simulink model "engine_approxdyn"  (Simulink 7.2)
settings: Solver=ode3  StartTime=0.0  StopTime=10.0  FixedStep=0.02  RelTol=1e-3
settings Model: Creator=E183308  LastModifiedBy=E183308

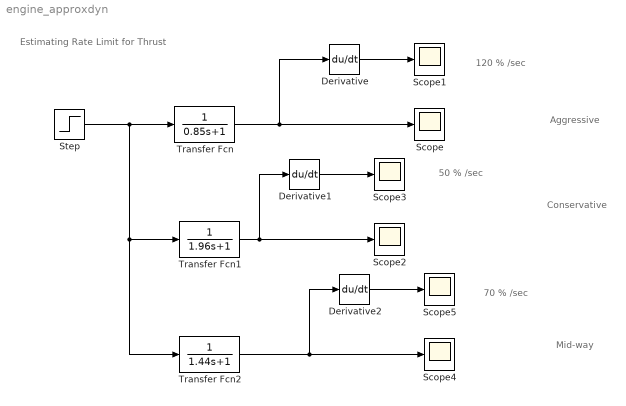
== system engine_approxdyn ==
  note: Conservative
  note: Estimating Rate Limit
      | for Thrust
  note: Aggressive
  note: Mid-way
  note: 120 % /sec
  note: 50 % /sec
  note: 70 % /sec
  Derivative : Derivative
  Derivative1 : Derivative
  Derivative2 : Derivative
  Scope{,1..5} (6 alike) : Scope
      Scope2 settings: SaveName=ScopeData2
      Scope3 settings: SaveName=ScopeData3
      Scope4 settings: SaveName=ScopeData4
      Scope5 settings: SaveName=ScopeData5
  Step : Step  After=100  SampleTime=0
  Transfer Fcn : TransferFcn  Denominator=[0.85 1]
  Transfer Fcn1 : TransferFcn  Denominator=[1.96 1]
  Transfer Fcn2 : TransferFcn  Denominator=[1.44 1]
  wires:
  Transfer Fcn/1 -> Derivative/1, Scope/1
  Derivative/1 -> Scope1/1
  Step/1 -> Transfer Fcn/1, Transfer Fcn1/1, Transfer Fcn2/1
  Transfer Fcn1/1 -> Scope2/1, Derivative1/1
  Derivative1/1 -> Scope3/1
  Transfer Fcn2/1 -> Derivative2/1, Scope4/1
  Derivative2/1 -> Scope5/1
